simulink model "Ejercicio2"  (R2015a)
settings: Solver=ode45  StartTime=0.0  StopTime=20  RelTol=1e-3
values from neighbouring files (symbols this model uses):
  C = Ch*inv(D)    [invhomo.m]
undefined symbols (not defined in the file or in its folder): L, R
settings Model: Creator=Alicia  LastModifiedBy=Alicia

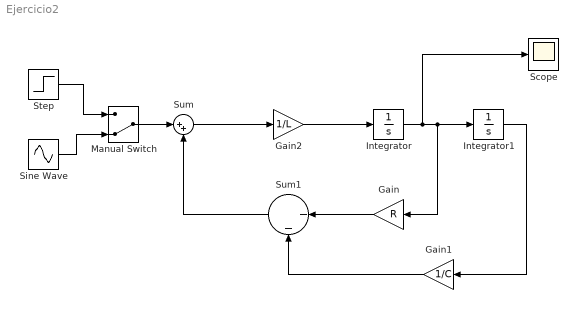
== system Ejercicio2 ==
  Gain : Gain  Gain=R
  Gain1 : Gain  Gain=1/C
  Gain2 : Gain  Gain=1/L
  Integrator : Integrator
  Integrator1 : Integrator
  Manual Switch : ManualSwitch  CurrentSetting=0
  Scope : Scope
      settings: TimeRange=1.787072243346007  YMin=-0.4  YMax=0.4
  Sine Wave : Sin  Amplitude=5  SampleTime=0
  Step : Step  Time=0  SampleTime=0
  Sum : Sum  Inputs=|++
  Sum1 : Sum  Inputs=|||-||-
  wires:
  Integrator/1 -> Scope/1, Gain/1, Integrator1/1
  Integrator1/1 -> Gain1/1
  Gain/1 -> Sum1/1
  Gain1/1 -> Sum1/2
  Sum1/1 -> Sum/2
  Sum/1 -> Gain2/1
  Gain2/1 -> Integrator/1
  Manual Switch/1 -> Sum/1
  Step/1 -> Manual Switch/1
  Sine Wave/1 -> Manual Switch/2
